simulink model "P_5_experimento_3"  (R2020b)
settings: Solver=VariableStepAuto  StartTime=0.0  StopTime=inf  RelTol=1e-3
undefined symbols (not defined in the file): serial
libraries: instrumentlib x2
settings Model: Creator=Brizz  LastModifiedBy=Brizz

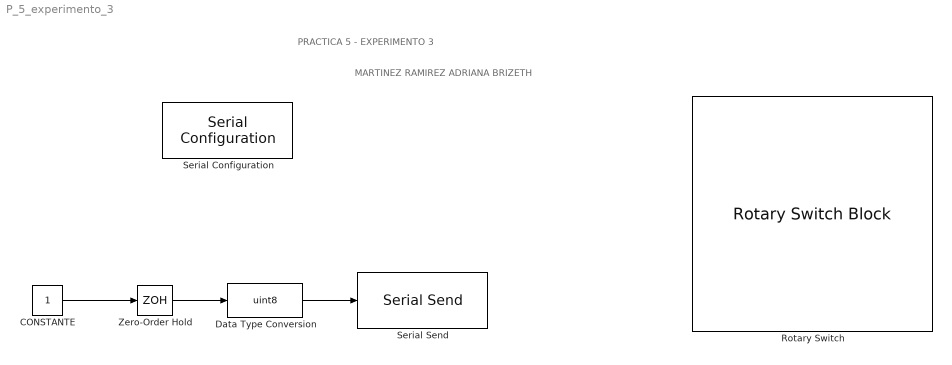
== system P_5_experimento_3 ==
  note: MARTINEZ RAMIREZ ADRIANA BRIZETH
  note: PRACTICA 5 - EXPERIMENTO 3
  CONSTANTE : Constant
  Data Type Conversion : DataTypeConversion  OutDataTypeStr=uint8
  Rotary Switch : RotarySwitchBlock
      settings: Values={{'0%', '10%', '20%', '30%', '40%', '50%', '60%', '70%', '80%', '90%', '100%', 'R', 'G', 'B'}, [1 10 20 30 40 50 60 70 80 90 100 82 86 65]}
  Serial Configuration : instrumentlib/Serial Configuration  Priority=-200000  ComPortMenu=COM5  ComPort=COM5  ObjConstructor=serial('COM5');  BaudRate=9600  DataBits=8  Parity=none  StopBits=1  FlowControl=none  Timeout=10  ByteOrder=LittleEndian
  Serial Send : instrumentlib/Serial Send  ComPortMenu=COM5  ComPort=COM5  ObjConstructor=serial('COM5');  Terminator=<none>  EnableBlockingMode=on
  Zero-Order Hold : ZeroOrderHold  SampleTime=0.5
  wires:
  CONSTANTE/1 -> Zero-Order Hold/1
  Zero-Order Hold/1 -> Data Type Conversion/1
  Data Type Conversion/1 -> Serial Send/1
